simulink model "SingleJoint_PID_Block"  (R2015b)
settings: Solver=VariableStepAuto  StartTime=0.0  StopTime=100  RelTol=1e-3
settings Model: Creator=wfxu  LastModifiedBy=wfxu

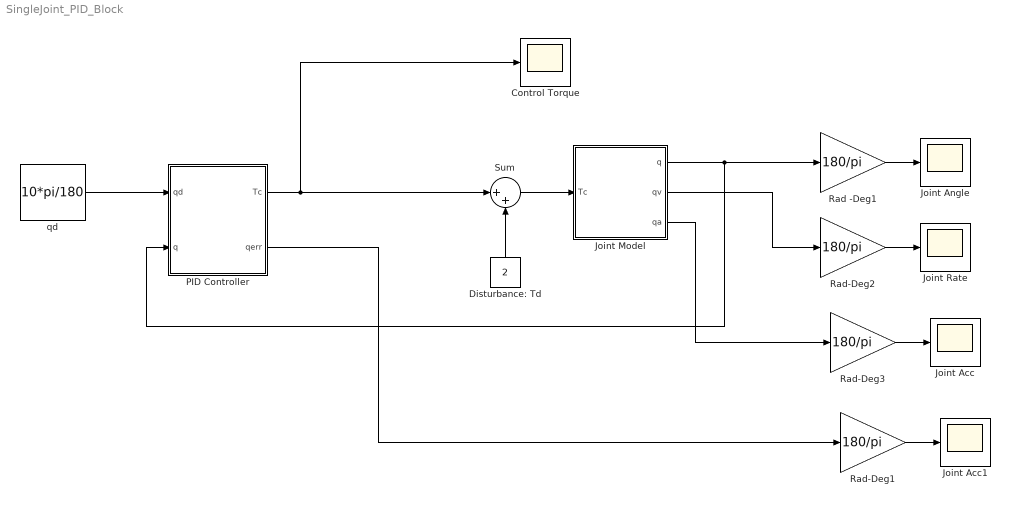
== system SingleJoint_PID_Block ==
  Control Torque : Scope
  Disturbance: Td : Constant  Value=2
  Joint Acc : Scope
  Joint Acc1 : Scope
  Joint Angle : Scope
  Joint Model : Subsystem
  Joint Rate : Scope
  "PID Controller " : Subsystem
  Rad -Deg1 : Gain  Gain=180/pi
  Rad-Deg1 : Gain  Gain=180/pi
  Rad-Deg2 : Gain  Gain=180/pi
  Rad-Deg3 : Gain  Gain=180/pi
  Sum : Sum  Inputs=|++
  qd : Constant  Value=10*pi/180
  wires:
  "PID Controller "/1(Tc) -> Sum/1, Control Torque/1
  Joint Model/1(q) -> Rad -Deg1/1, "PID Controller "/2(q)
  qd/1 -> "PID Controller "/1(qd)
  Disturbance: Td/1 -> Sum/2
  Sum/1 -> Joint Model/1(Tc)
  Rad-Deg3/1 -> Joint Acc/1
  Rad -Deg1/1 -> Joint Angle/1
  Rad-Deg2/1 -> Joint Rate/1
  Joint Model/2(qv) -> Rad-Deg2/1
  Joint Model/3(qa) -> Rad-Deg3/1
  Rad-Deg1/1 -> Joint Acc1/1
  "PID Controller "/2(qerr) -> Rad-Deg1/1

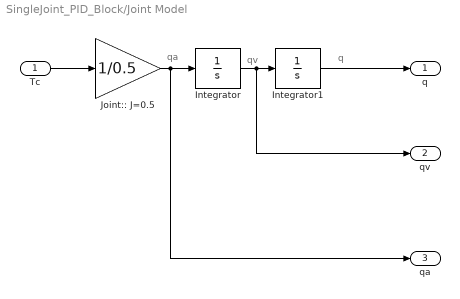
== system SingleJoint_PID_Block/Joint Model ==
  note: qa
  note: qv
  note: q
  Tc : Inport
  Integrator : Integrator
  Integrator1 : Integrator
  Joint:: J=0.5 : Gain  Gain=1/0.5
  q : Outport
  qv : Outport  Port=2
  qa : Outport  Port=3
  wires:
  Integrator1/1 -> q/1
  Integrator/1 -> qv/1, Integrator1/1
  Joint:: J=0.5/1 -> qa/1, Integrator/1
  Tc/1 -> Joint:: J=0.5/1

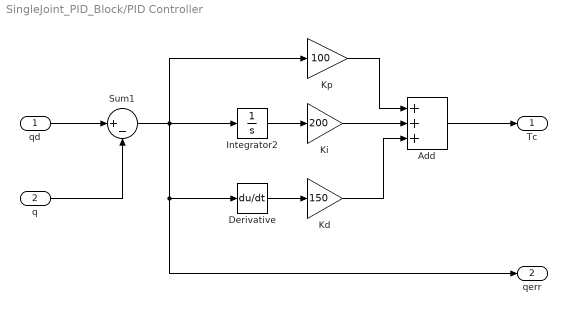
== system SingleJoint_PID_Block/PID Controller  ==
  qd : Inport
  q : Inport  Port=2
  Add : Sum  Inputs=+++
  Derivative : Derivative
  Integrator2 : Integrator
  Kd : Gain  Gain=150
  Ki : Gain  Gain=200
  Kp : Gain  Gain=100
  Sum1 : Sum  Inputs=|+-
  Tc : Outport
  qerr : Outport  Port=2
  wires:
  Kd/1 -> Add/3
  Ki/1 -> Add/2
  Add/1 -> Tc/1
  Integrator2/1 -> Ki/1
  Kp/1 -> Add/1
  Derivative/1 -> Kd/1
  qd/1 -> Sum1/1
  q/1 -> Sum1/2
  Sum1/1 -> qerr/1, Derivative/1, Kp/1, Integrator2/1
